simulink model "sim_ForgetMRE_case4"  (R2023a)
settings: Solver=ode3  StartTime=0.0  StopTime=150  FixedStep=Ts  MaxStep=Ts  RelTol=1e-4
values from neighbouring files (symbols this model uses):
  b0 = 30    [Initial_par.m]
  b1 = 11    [Initial_par.m]
  c1 = 1    [Initial_par.m]
  c2 = 1    [Initial_par.m]
  c3 = 1    [Initial_par.m]
  gamma = 1    [Initial_par.m]
  kpa = [kap1,kap2,kap3]    [Initial_par.m]
  lambda = 1    [Initial_par.m]
  N = 3    [Initial_par.m]
  th = [0.4,0.5,0.1]'    [Initial_par.m]
  Ts = 1e-3    (= 0.001)    [Initial_par.m]
  vari = SD^2    (= 1e-06)    [Initial_par.m]
  x0 = [0,0,0]'    [Initial_par.m]    (also in TO_sys.m = x_init)
  zeta0 = -z0    [Initial_par.m]
undefined symbols (not defined in the file or in its folder): Phi0, z0
libraries: matrix_library x6
settings Model: Creator=stt  LastModifiedBy=stt
settings SolverCC: SolverResetMethod=Robust
settings OptimizationCC: ReuseModelBlockBuffer=off

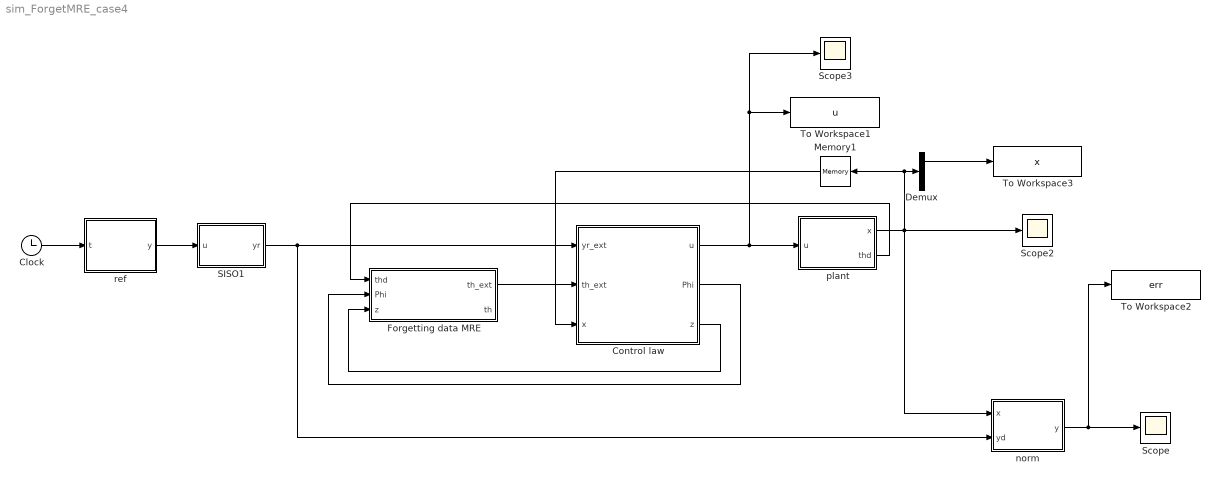
== system sim_ForgetMRE_case4 ==
  Clock : Clock
  Control law : Subsystem
  Demux : Demux  Outputs=3
  Forgetting data MRE : Subsystem
  Memory1 : Memory  InitialCondition=x0
  SISO1 : Subsystem
  Scope : Scope
  Scope2 : Scope
  Scope3 : Scope
  To Workspace1 : ToWorkspace  VariableName=u  SaveFormat=Timeseries  SampleTime=-1
  To Workspace2 : ToWorkspace  VariableName=err  SaveFormat=Timeseries  SampleTime=-1
  To Workspace3 : ToWorkspace  VariableName=x  SaveFormat=Timeseries  SampleTime=-1
  norm : MATLAB Function  TreatAsAtomicUnit=on
  plant : Subsystem
  ref : MATLAB Function  TreatAsAtomicUnit=on
  wires:
  ref/1(y) -> SISO1/1(u)
  norm/1(y) -> To Workspace2/1, Scope/1
  plant/1(x) -> Demux/1, Memory1/1, norm/1(x), Scope2/1
  Demux/1 -> To Workspace3/1
  Clock/1 -> ref/1(t)
  Control law/2(Phi) -> Forgetting data MRE/2(Phi)
  Control law/1(u) -> To Workspace1/1, Scope3/1, plant/1(u)
  Memory1/1 -> Control law/3(x)
  Forgetting data MRE/1(th_ext) -> Control law/2(th_ext)
  Control law/3(z) -> Forgetting data MRE/3(z)
  plant/2(thd) -> Forgetting data MRE/1(thd)
  SISO1/1(yr) -> norm/2(yd), Control law/1(yr_ext)

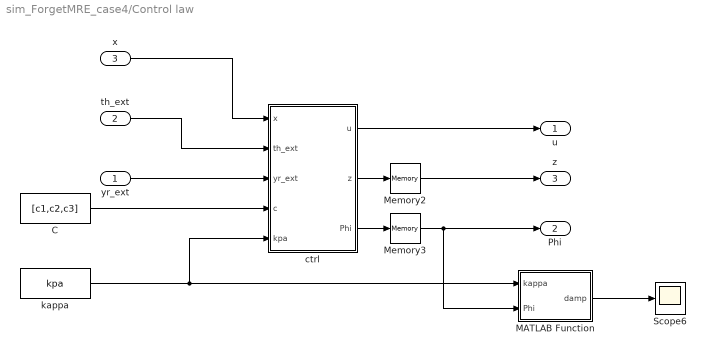
== system sim_ForgetMRE_case4/Control law ==
  yr_ext : Inport
  th_ext : Inport  Port=2
  x : Inport  Port=3
  C : Constant  Value=[c1,c2,c3]
  MATLAB Function : MATLAB Function  TreatAsAtomicUnit=on
  Memory2 : Memory  InitialCondition=z0
  Memory3 : Memory  InitialCondition=Phi0
  Scope6 : Scope
  ctrl : MATLAB Function  TreatAsAtomicUnit=on
  kappa : Constant  Value=kpa
  u : Outport
  Phi : Outport  Port=2
  z : Outport  Port=3
  wires:
  ctrl/3(Phi) -> Memory3/1
  Memory3/1 -> MATLAB Function/2(Phi), Phi/1
  th_ext/1 -> ctrl/2(th_ext)
  kappa/1 -> ctrl/5(kpa), MATLAB Function/1(kappa)
  C/1 -> ctrl/4(c)
  Memory2/1 -> z/1
  ctrl/2(z) -> Memory2/1
  yr_ext/1 -> ctrl/3(yr_ext)
  x/1 -> ctrl/1(x)
  ctrl/1(u) -> u/1
  MATLAB Function/1(damp) -> Scope6/1

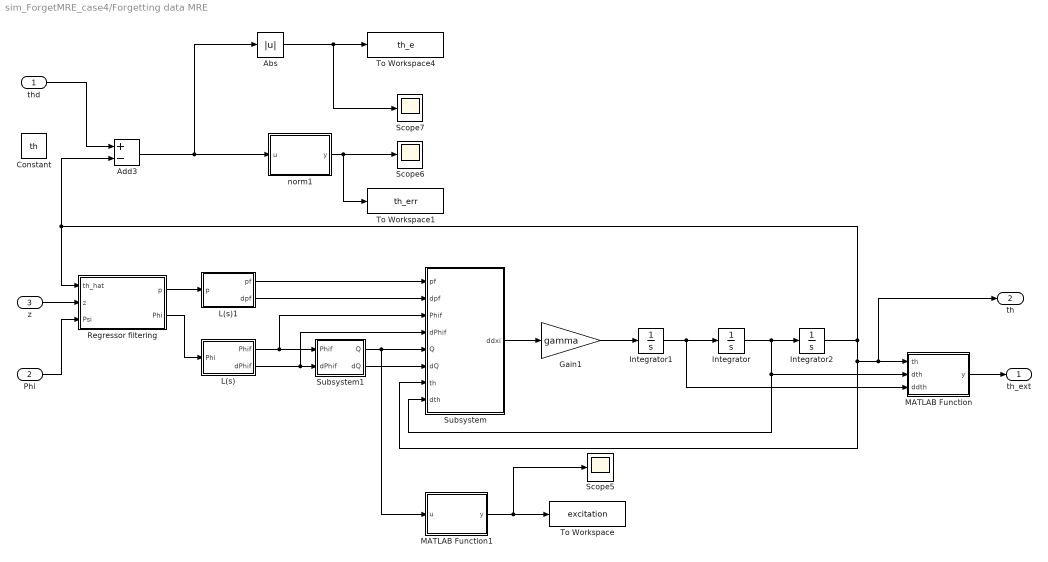
== system sim_ForgetMRE_case4/Forgetting data MRE ==
  thd : Inport
  Phi : Inport  Port=2
  z : Inport  Port=3
  Abs : Abs  SaturateOnIntegerOverflow=off
  Add3 : Sum  Inputs=+-
  Constant : Constant  Value=th
  Gain1 : Gain  Gain=gamma
  Integrator : Integrator  InitialCondition=zeros(N,1)
  Integrator1 : Integrator  InitialCondition=zeros(N,1)
  Integrator2 : Integrator  InitialCondition=zeros(N,1)
  L(s) : Subsystem
  L(s)1 : Subsystem
  MATLAB Function : MATLAB Function  TreatAsAtomicUnit=on
  MATLAB Function1 : MATLAB Function  TreatAsAtomicUnit=on
  Regressor filtering : Subsystem
  Scope5 : Scope
  Scope6 : Scope
  Scope7 : Scope
  Subsystem : Subsystem
  Subsystem1 : Subsystem
  To Workspace : ToWorkspace  VariableName=excitation  SaveFormat=Timeseries  SampleTime=-1
  To Workspace1 : ToWorkspace  VariableName=th_err  SaveFormat=Timeseries  SampleTime=-1
  To Workspace4 : ToWorkspace  VariableName=th_e  SaveFormat=Timeseries  SampleTime=-1
  norm1 : MATLAB Function  TreatAsAtomicUnit=on
  th_ext : Outport
  th : Outport  Port=2
  wires:
  MATLAB Function/1(y) -> th_ext/1
  MATLAB Function1/1(y) -> Scope5/1, To Workspace/1
  norm1/1(y) -> Scope6/1, To Workspace1/1
  thd/1 -> Add3/1
  Add3/1 -> Abs/1, norm1/1(u)
  Regressor filtering/2(Phi) -> L(s)/1(Phi)
  Regressor filtering/1(p) -> L(s)1/1(p)
  z/1 -> Regressor filtering/2(z)
  Phi/1 -> Regressor filtering/3(Psi)
  L(s)1/2(dpf) -> Subsystem/2(dpf)
  L(s)1/1(pf) -> Subsystem/1(pf)
  L(s)/1(Phif) -> Subsystem1/1(Phif), Subsystem/3(Phif)
  L(s)/2(dPhif) -> Subsystem1/2(dPhif), Subsystem/4(dPhif)
  Subsystem1/1(Q) -> MATLAB Function1/1(u), Subsystem/5(Q)
  Subsystem1/2(dQ) -> Subsystem/6(dQ)
  Subsystem/1(ddxi) -> Gain1/1
  Gain1/1 -> Integrator1/1
  Integrator1/1 -> MATLAB Function/3(ddth), Integrator/1
  Integrator2/1 -> th/1, MATLAB Function/1(th), Subsystem/7(th), Regressor filtering/1(th_hat), Add3/2
  Integrator/1 -> Subsystem/8(dth), MATLAB Function/2(dth), Integrator2/1
  Abs/1 -> Scope7/1, To Workspace4/1

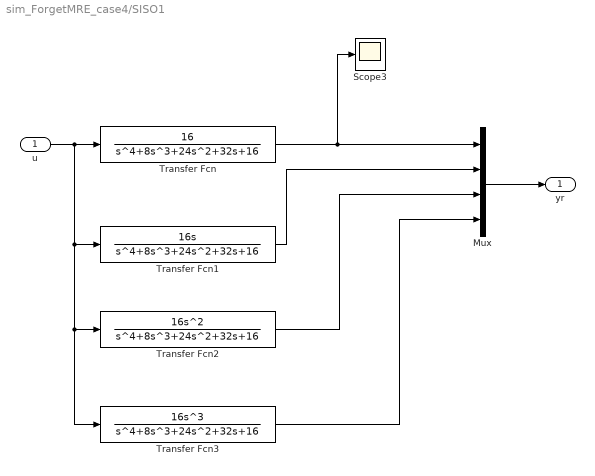
== system sim_ForgetMRE_case4/SISO1 ==
  u : Inport
  Mux : Mux
  Scope3 : Scope
  Transfer Fcn : TransferFcn  Numerator=[16]  Denominator=[1 8 24 32 16]
  Transfer Fcn1 : TransferFcn  Numerator=[16 0]  Denominator=[1 8 24 32 16]
  Transfer Fcn2 : TransferFcn  Numerator=[16 0 0]  Denominator=[1 8 24 32 16]
  Transfer Fcn3 : TransferFcn  Numerator=[16 0 0 0]  Denominator=[1 8 24 32 16]
  yr : Outport
  wires:
  u/1 -> Transfer Fcn3/1, Transfer Fcn2/1, Transfer Fcn1/1, Transfer Fcn/1
  Transfer Fcn/1 -> Scope3/1, Mux/1
  Transfer Fcn1/1 -> Mux/2
  Transfer Fcn2/1 -> Mux/3
  Transfer Fcn3/1 -> Mux/4
  Mux/1 -> yr/1

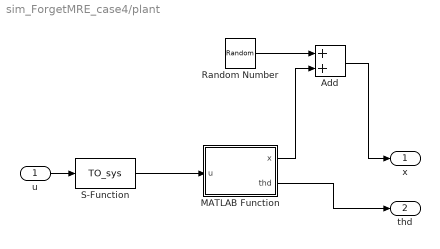
== system sim_ForgetMRE_case4/plant ==
  u : Inport
  Add : Sum
  MATLAB Function : MATLAB Function  TreatAsAtomicUnit=on
  Random Number : RandomNumber  Variance=vari  SampleTime=Ts
  S-Function : S-Function  FunctionName=TO_sys  Parameters=x0,th  SFunctionDeploymentMode=off  EnableBusSupport=off
  x : Outport
  thd : Outport  Port=2
  wires:
  u/1 -> S-Function/1
  S-Function/1 -> MATLAB Function/1(u)
  Add/1 -> x/1
  MATLAB Function/2(thd) -> thd/1
  MATLAB Function/1(x) -> Add/2
  Random Number/1 -> Add/1

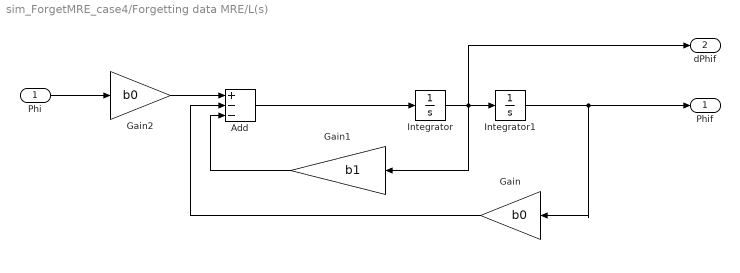
== system sim_ForgetMRE_case4/Forgetting data MRE/L(s) ==
  Phi : Inport
  Add : Sum  Inputs=+--
  Gain : Gain  Gain=b0
  Gain1 : Gain  Gain=b1
  Gain2 : Gain  Gain=b0
  Integrator : Integrator
  Integrator1 : Integrator
  Phif : Outport
  dPhif : Outport  Port=2
  wires:
  Phi/1 -> Gain2/1
  Integrator1/1 -> Gain/1, Phif/1
  Add/1 -> Integrator/1
  Integrator/1 -> Gain1/1, dPhif/1, Integrator1/1
  Gain1/1 -> Add/3
  Gain/1 -> Add/2
  Gain2/1 -> Add/1

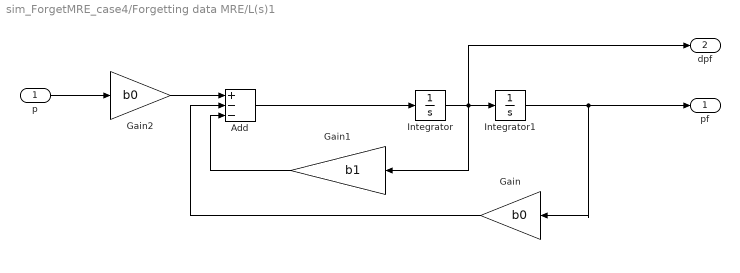
== system sim_ForgetMRE_case4/Forgetting data MRE/L(s)1 ==
  p : Inport
  Add : Sum  Inputs=+--
  Gain : Gain  Gain=b0
  Gain1 : Gain  Gain=b1
  Gain2 : Gain  Gain=b0
  Integrator : Integrator
  Integrator1 : Integrator
  pf : Outport
  dpf : Outport  Port=2
  wires:
  p/1 -> Gain2/1
  Integrator1/1 -> Gain/1, pf/1
  Add/1 -> Integrator/1
  Integrator/1 -> Gain1/1, dpf/1, Integrator1/1
  Gain1/1 -> Add/3
  Gain/1 -> Add/2
  Gain2/1 -> Add/1

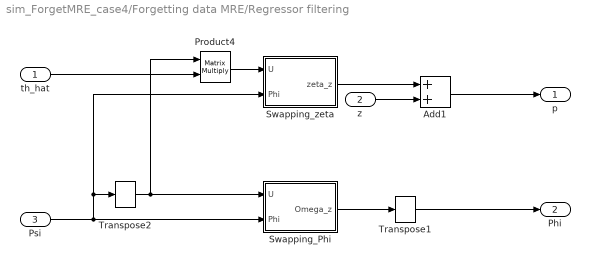
== system sim_ForgetMRE_case4/Forgetting data MRE/Regressor filtering ==
  th_hat : Inport
  z : Inport  Port=2
  Psi : Inport  Port=3
  Add1 : Sum
  Product4 : Product  Multiplication=Matrix(*)
  Swapping_Phi : Subsystem
  Swapping_zeta : Subsystem
  Transpose1 : matrix_library/Transpose
  Transpose2 : matrix_library/Transpose
  p : Outport
  Phi : Outport  Port=2
  wires:
  Product4/1 -> Swapping_zeta/1(U)
  th_hat/1 -> Product4/2
  Psi/1 -> Swapping_Phi/2(Phi), Swapping_zeta/2(Phi), Transpose2/1
  Swapping_zeta/1(zeta_z) -> Add1/1
  Transpose2/1 -> Swapping_Phi/1(U), Product4/1
  z/1 -> Add1/2
  Add1/1 -> p/1
  Swapping_Phi/1(Omega_z) -> Transpose1/1
  Transpose1/1 -> Phi/1

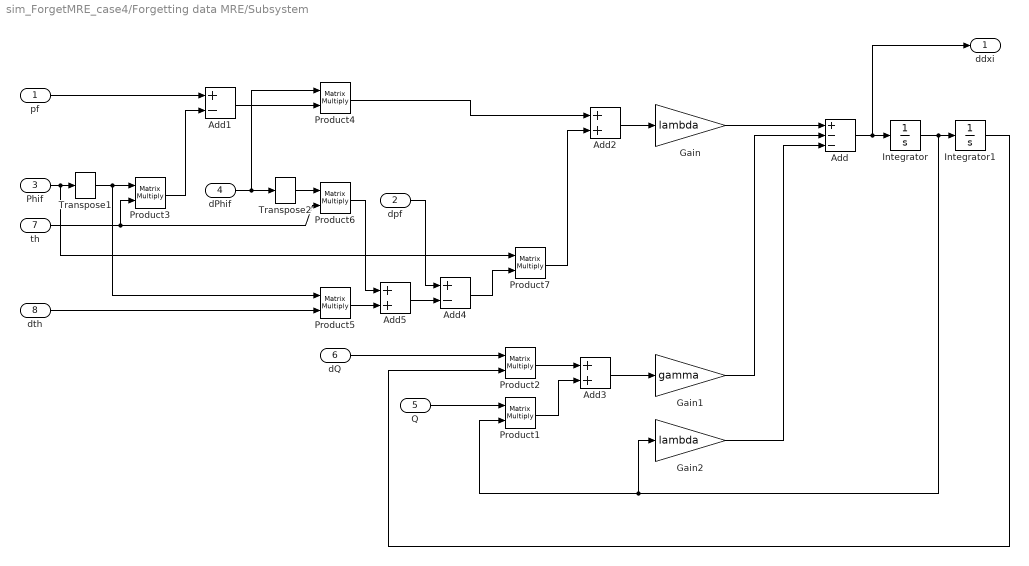
== system sim_ForgetMRE_case4/Forgetting data MRE/Subsystem ==
  pf : Inport
  dpf : Inport  Port=2
  Phif : Inport  Port=3
  dPhif : Inport  Port=4
  Q : Inport  Port=5
  dQ : Inport  Port=6
  th : Inport  Port=7
  dth : Inport  Port=8
  Add : Sum  Inputs=+--
  Add1 : Sum  Inputs=+-
  Add2 : Sum
  Add3 : Sum
  Add4 : Sum  Inputs=+-
  Add5 : Sum
  Gain : Gain  Gain=lambda
  Gain1 : Gain  Gain=gamma
  Gain2 : Gain  Gain=lambda
  Integrator : Integrator  InitialCondition=zeros(N,1)
  Integrator1 : Integrator  InitialCondition=zeros(N,1)
  Product{1..7} (7 alike) : Product  Multiplication=Matrix(*)
  Transpose1 : matrix_library/Transpose
  Transpose2 : matrix_library/Transpose
  ddxi : Outport
  wires:
  Q/1 -> Product1/1
  dQ/1 -> Product2/1
  Product1/1 -> Add3/2
  Add3/1 -> Gain1/1
  pf/1 -> Add1/1
  Product3/1 -> Add1/2
  Phif/1 -> Product7/1, Transpose1/1
  Transpose1/1 -> Product3/1, Product5/1
  th/1 -> Product6/2, Product3/2
  Add1/1 -> Product4/2
  dPhif/1 -> Product4/1, Transpose2/1
  Product4/1 -> Add2/1
  dpf/1 -> Add4/1
  dth/1 -> Product5/2
  Transpose2/1 -> Product6/1
  Product5/1 -> Add5/2
  Product6/1 -> Add5/1
  Add5/1 -> Add4/2
  Add4/1 -> Product7/2
  Product7/1 -> Add2/2
  Add2/1 -> Gain/1
  Gain/1 -> Add/1
  Gain1/1 -> Add/2
  Add/1 -> ddxi/1, Integrator/1
  Integrator/1 -> Gain2/1, Product1/2, Integrator1/1
  Gain2/1 -> Add/3
  Integrator1/1 -> Product2/2
  Product2/1 -> Add3/1

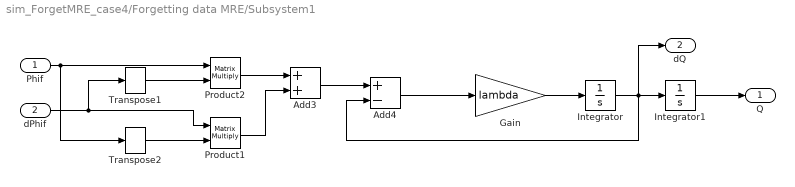
== system sim_ForgetMRE_case4/Forgetting data MRE/Subsystem1 ==
  Phif : Inport
  dPhif : Inport  Port=2
  Add3 : Sum
  Add4 : Sum  Inputs=+-
  Gain : Gain  Gain=lambda
  Integrator : Integrator
  Integrator1 : Integrator
  Product1 : Product  Multiplication=Matrix(*)
  Product2 : Product  Multiplication=Matrix(*)
  Transpose1 : matrix_library/Transpose
  Transpose2 : matrix_library/Transpose
  Q : Outport
  dQ : Outport  Port=2
  wires:
  Phif/1 -> Product2/1, Transpose2/1
  dPhif/1 -> Product1/1, Transpose1/1
  Product1/1 -> Add3/2
  Transpose1/1 -> Product2/2
  Transpose2/1 -> Product1/2
  Product2/1 -> Add3/1
  Add4/1 -> Gain/1
  Add3/1 -> Add4/1
  Gain/1 -> Integrator/1
  Integrator/1 -> Add4/2, dQ/1, Integrator1/1
  Integrator1/1 -> Q/1

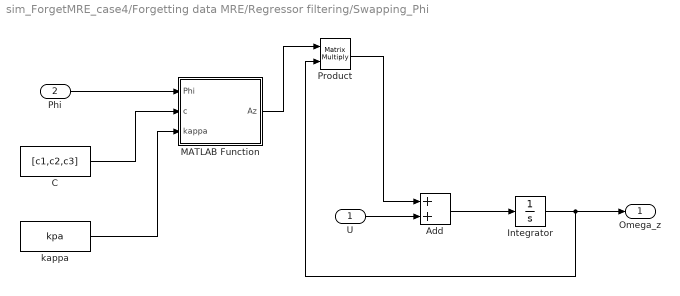
== system sim_ForgetMRE_case4/Forgetting data MRE/Regressor filtering/Swapping_Phi ==
  U : Inport
  Phi : Inport  Port=2
  Add : Sum
  C : Constant  Value=[c1,c2,c3]
  Integrator : Integrator
  MATLAB Function : MATLAB Function  TreatAsAtomicUnit=on
  Product : Product  Multiplication=Matrix(*)
  kappa : Constant  Value=kpa
  Omega_z : Outport
  wires:
  Phi/1 -> MATLAB Function/1(Phi)
  C/1 -> MATLAB Function/2(c)
  kappa/1 -> MATLAB Function/3(kappa)
  MATLAB Function/1(Az) -> Product/1
  Product/1 -> Add/1
  Add/1 -> Integrator/1
  U/1 -> Add/2
  Integrator/1 -> Product/2, Omega_z/1

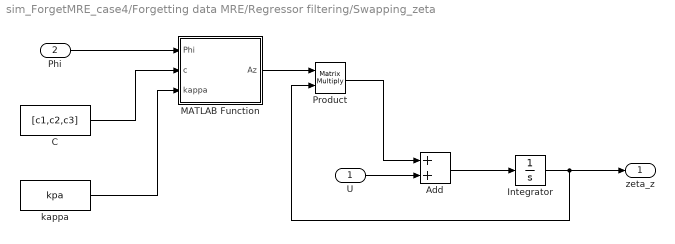
== system sim_ForgetMRE_case4/Forgetting data MRE/Regressor filtering/Swapping_zeta ==
  U : Inport
  Phi : Inport  Port=2
  Add : Sum
  C : Constant  Value=[c1,c2,c3]
  Integrator : Integrator  InitialCondition=zeta0
  MATLAB Function : MATLAB Function  TreatAsAtomicUnit=on
  Product : Product  Multiplication=Matrix(*)
  kappa : Constant  Value=kpa
  zeta_z : Outport
  wires:
  Phi/1 -> MATLAB Function/1(Phi)
  C/1 -> MATLAB Function/2(c)
  kappa/1 -> MATLAB Function/3(kappa)
  MATLAB Function/1(Az) -> Product/1
  Product/1 -> Add/1
  Add/1 -> Integrator/1
  U/1 -> Add/2
  Integrator/1 -> Product/2, zeta_z/1

== matlab function sim_ForgetMRE_case4/Control law/ctrl ==
  data: x input; th_ext input; yr_ext input; u output; c input; kpa input; z output; Phi output
function [u,z,Phi] = fcn(x,th_ext,yr_ext,c,kpa)



[alpha1,alpha2,u,z,Phi]=virtual_ctrl(x,th_ext,yr_ext,kpa,c);
vir_u=[alpha1,alpha2];

== matlab function sim_ForgetMRE_case4/Forgetting data MRE/MATLAB Function1 ==
  data: u input; y output
function y = fcn(u)

y = min(svd(u));

== matlab function sim_ForgetMRE_case4/ref ==
  data: t input; y output
function y = fcn(t)

if t<10
    y=0.2;
% elseif t<80
    % y=-0.5;
% elseif t<50
%     y=0.5;
else
    y=-1.5;
end


% A=1;T=1;
% y=[A*sin(T*t);A*T*cos(T*t);-A*T*T*sin(T*t);-A*T*T*T*cos(T*t)];
% y=1.2*sin(0.8*t)+0.8*cos(0.4*t)-0.8;

== matlab function sim_ForgetMRE_case4/norm ==
  data: x input; y output; yd input
function y= fcn(x,yd)
err=x(1)-yd(1);
y = abs(err);

== matlab function sim_ForgetMRE_case4/Forgetting data MRE/Regressor filtering/Swapping_zeta/MATLAB Function ==
  data: Phi input; Az output; c input; kappa input
function Az = fcn(Phi,c,kappa)
c1=c(1);c2=c(2);c3=c(3);
kap1=kappa(1);kap2=kappa(2);kap3=kappa(3);
phi1=Phi(:,1);phi2=Phi(:,2);phi3=Phi(:,3);
Dg=-[c1+kap1*norm(phi1)^2,c2+kap2*norm(phi2)^2,c3+kap3*norm(phi3)^2];
Az=diag(Dg)+diag([1,1],1)-diag([1,1],-1);

== matlab function sim_ForgetMRE_case4/Forgetting data MRE/Regressor filtering/Swapping_Phi/MATLAB Function ==
  data: Phi input; Az output; c input; kappa input
function Az = fcn(Phi,c,kappa)
c1=c(1);c2=c(2);c3=c(3);
kap1=kappa(1);kap2=kappa(2);kap3=kappa(3);
phi1=Phi(:,1);phi2=Phi(:,2);phi3=Phi(:,3);
Dg=-[c1+kap1*norm(phi1)^2,c2+kap2*norm(phi2)^2,c3+kap3*norm(phi3)^2];
Az=diag(Dg)+diag([1,1],1)-diag([1,1],-1);

== matlab function sim_ForgetMRE_case4/plant/MATLAB Function ==
  data: u input; x output; thd output
function [x,thd] = fcn(u)

x=u(1:3);
thd=u(4:6);

== matlab function sim_ForgetMRE_case4/Forgetting data MRE/MATLAB Function ==
  data: th input; y output; dth input; ddth input
function y = fcn(th,dth,ddth)

y = [th,dth,ddth];

== matlab function sim_ForgetMRE_case4/Forgetting data MRE/norm1 ==
  data: u input; y output
function y = fcn(u)

y = norm(u);

== matlab function sim_ForgetMRE_case4/Control law/MATLAB Function ==
  data: kappa input; damp output; Phi input
function damp = fcn(kappa,Phi)
kap1=kappa(1);kap2=kappa(2);kap3=kappa(3);
phi1=Phi(:,1);phi2=Phi(:,2);phi3=Phi(:,3);
damp=-[kap1*norm(phi1)^2,kap2*norm(phi2)^2,kap3*norm(phi3)^2];
